simulink model "gm_Watermarker_vnl"  (R2022a)
settings: Solver=FixedStepDiscrete  StartTime=0.0  StopTime=256*256-1  RelTol=1e-3
undefined symbols (not defined in the file or in its folder): alpha, T0, T1
libraries: hdlsllib x20, simulink x2, dspsrcs4 x2
Description:
  | Performs watermarking.
  | In:
  | - One channel of 8-bit image 256x256
  | - Watermark (64 bits)
  | Out:
  | - Watermarked image channel
settings Model: SimulationMode=accelerator  Creator=The MathWorks, Inc.  LastModifiedBy=Администратор
settings SolverCC: AlgebraicLoopSolver=TrustRegion
settings DataIOCC: LimitDataPoints=on  SaveFormat=Structure  SaveTime=off  ReturnWorkspaceOutputs=off
settings OptimizationCC: BlockReduction=off  ConditionallyExecuteInputs=off  DefaultParameterBehavior=Inlined  InheritOutputTypeSmallerThanSingle=on  LifeSpan=inf
settings DebuggingCC: AlgebraicLoopMsg=error  UnderspecifiedInitializationDetection=Classic  MergeDetectMultiDrivingBlocksExec=none  SolverPrmCheckMsg=warning  InheritedTsInSrcMsg=none  SingleTaskRateTransMsg=error  ParameterPrecisionLossMsg=none  UnconnectedInputMsg=warning  UnconnectedOutputMsg=warning  UnconnectedLineMsg=warning  AllowSymbolicDim=off  SFUnexpectedBacktrackingDiag=warning  SFNoUnconditionalDefaultTransitionDiag=warning  SFExecutionAtInitializationDiag=none  SFMachineParentedDataDiag=warning  ArithmeticOperatorsInVariantConditions=warning
settings HardwareCC: ProdBitPerPointer=32  ProdBitPerSizeT=32  ProdBitPerPtrDiffT=32  ProdLargestAtomicFloat=None  ProdIntDivRoundTo=Undefined  ProdEndianess=Unspecified  ProdWordSize=32  ProdHWDeviceType=ASIC/FPGA->ASIC/FPGA  TargetBitPerPointer=64  TargetBitPerSizeT=64  TargetBitPerPtrDiffT=64  TargetLongLongMode=on  TargetIntDivRoundTo=Zero  TargetEndianess=LittleEndian  TargetWordSize=64  TargetHWDeviceType=Custom Processor->MATLAB Host Computer  ProdEqTarget=off
settings ModelReferenceCC: PropagateSignalLabelsOutOfModel=off
settings SFSimCC: SimUseLocalCustomCode=off  CustomCodeUndefinedFunction=UseInterfaceOnly
settings RTWCC: RTWUseLocalCustomCode=off  DLArmComputeVersion=19.05
settings CodeAppCC: StateflowObjectComments=on
settings GRTTargetCC: TargetLangStandard=C89/C90 (ANSI)
settings ConfigComp: CovMetricSettings=dw  CovSaveCumulativeToWorkspaceVar=on  CovSaveSingleToWorkspaceVar=on  CovExternalEMLEnable=off  CovSFcnEnable=off

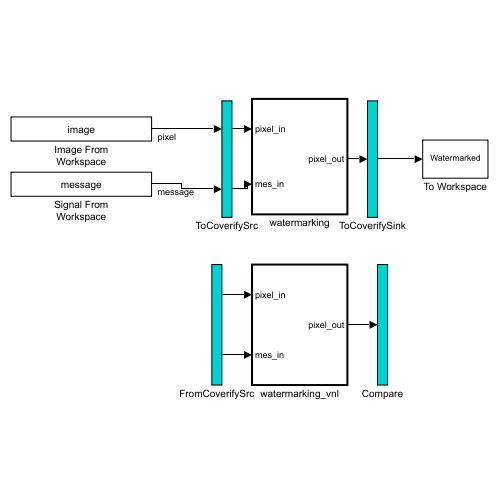
[thumbnail: Simulink's stored preview of the top-level diagram]
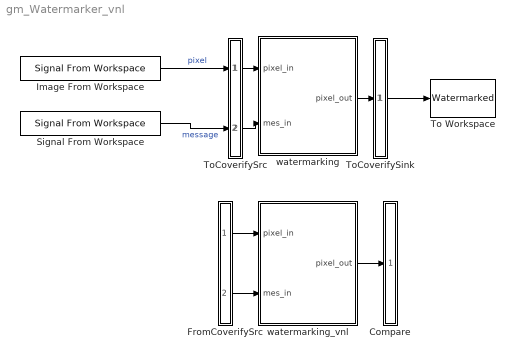
== system gm_Watermarker_vnl ==
  Compare : Subsystem
      mask Display: disp('')
  FromCoverifySrc : Subsystem
      mask Display: disp('')
  Image From Workspace : dspsrcs4/Signal From Workspace  X=image  Ts=1  nsamps=1  OutputAfterFinalValue=Cyclic repetition  ignoreOrWarnInputAndFrameLengths=off  OutputFrames=off
  Signal From Workspace : dspsrcs4/Signal From Workspace  X=message  Ts=1  nsamps=1  OutputAfterFinalValue=Cyclic repetition  ignoreOrWarnInputAndFrameLengths=off  OutputFrames=off
  To Workspace : ToWorkspace  VariableName=Watermarked  SampleTime=-1
      settings: Save2DSignal=2-D array (concatenate along first dimension)
  ToCoverifySink : Subsystem
      mask Display: disp('')
  ToCoverifySrc : Subsystem
      mask Display: disp('')
  watermarking : Subsystem  TreatAsAtomicUnit=on
  watermarking_vnl : Subsystem  TreatAsAtomicUnit=on
  wires:
  ToCoverifySrc/1(out1) -> watermarking/1(pixel_in)
  ToCoverifySrc/2(out2) -> watermarking/2(mes_in)
  watermarking/1(pixel_out) -> ToCoverifySink/1(in1)
  Image From Workspace/1 -> ToCoverifySrc/1(in1)  "pixel"
  Signal From Workspace/1 -> ToCoverifySrc/2(in2)  "message"
  ToCoverifySink/1(out1) -> To Workspace/1
  FromCoverifySrc/1(out1) -> watermarking_vnl/1(pixel_in)
  FromCoverifySrc/2(out2) -> watermarking_vnl/2(mes_in)
  watermarking_vnl/1(pixel_out) -> Compare/1(in1)

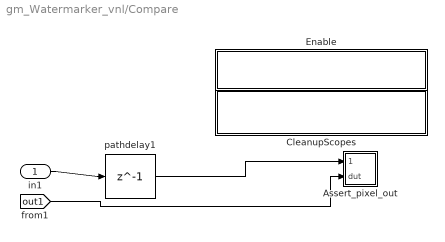
== system gm_Watermarker_vnl/Compare ==
  in1 : Inport
  Assert_pixel_out : Subsystem
  CleanupScopes : Subsystem
      settings: OpenFcn=|
      | blkName = gcb; %self block
      | idx = regexp(blkName, '/CleanupScopes$', 'once');
      | blkParent = blkName(1:idx-1);
      | blks=find_system(blkParent, 'LookUnderMasks', 'all','blocktype', 'Scope');
      | for itr = 1:length(blks)
      | 	 hScopeCfg = get_param(blks{itr},'ScopeConfiguration');
      | 	 hScopeCfg.Visible = ~ hScopeCfg.Visible;
      | end
      | drawnow;
      mask Display: fprintf(message('hdlcoder:cosim:vnl_dblclick').getString());
  Enable : Subsystem
      settings: OpenFcn=|
      | blkName = gcb;
      | idx = regexp(blkName, '/Enable$', 'once');
      | blkParent = blkName(1:idx-1);
      | blks=find_system(blkParent, 'LookUnderMasks', 'all','blocktype', 'Assertion');
      | e = get_param(blks{1}, 'Enabled');
      | if strcmp(e, 'on'), f= 'off';, else, f = 'on';, end
      | for ii=1:length(blks), set_param(blks{ii}, 'Enabled', f);, end
      | set_param(gcb, 'MaskDisplay',['fprintf(message(''hdlcoder:cosim:vnl_dblclick_assertions'',','''',upper(e),'''',').getString())']);
      mask Display: fprintf(message('hdlcoder:cosim:vnl_dblclick_assertions','OFF').getString());
  pathdelay1 : Delay  DelayLength=1
  wires:
  in1/1 -> pathdelay1/1
  pathdelay1/1 -> Assert_pixel_out/1(cosim)
  [out1] -> Assert_pixel_out/2(dut)

== system gm_Watermarker_vnl/FromCoverifySrc ==
  out1 : Outport
  out2 : Outport  Port=2
  wires:
  [in1] -> out1/1
  [in2] -> out2/1

== system gm_Watermarker_vnl/ToCoverifySink ==
  in1 : Inport
  out1 : Outport
  tag scope: out1=global
  wires:
  in1/1 -> out1/1, [out1]

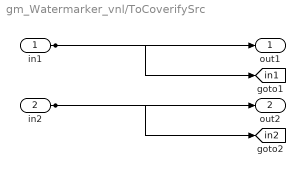
== system gm_Watermarker_vnl/ToCoverifySrc ==
  in1 : Inport
  in2 : Inport  Port=2
  out1 : Outport
  out2 : Outport  Port=2
  tag scope: in1=global, in2=global
  wires:
  in1/1 -> out1/1, [in1]
  in2/1 -> out2/1, [in2]

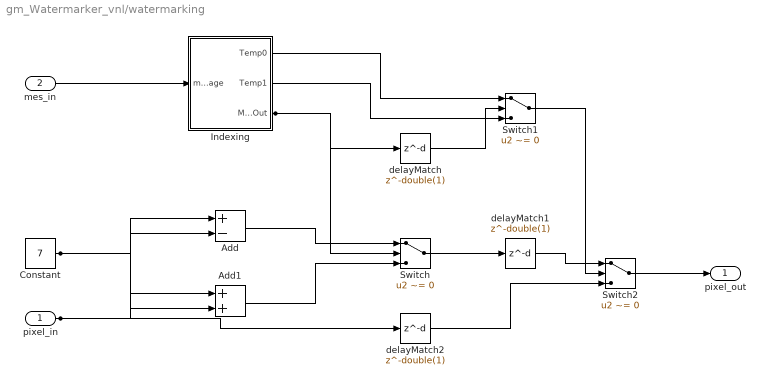
== system gm_Watermarker_vnl/watermarking ==
  pixel_in : Inport  OutDataTypeStr=uint8  PortDimensions=1  SampleTime=1
  mes_in : Inport  Port=2  OutDataTypeStr=boolean  PortDimensions=1  SampleTime=1
  Add : Sum  Inputs=+-  AccumDataTypeStr=uint8  OutDataTypeStr=uint8  SampleTime=1
  Add1 : Sum  AccumDataTypeStr=uint8  OutDataTypeStr=uint8  SampleTime=1
  Constant : Constant  Value=7  OutDataTypeStr=uint8  SampleTime=1
  Indexing : Subsystem
  Switch : Switch  Criteria=u2 ~= 0  Threshold=double(0)  OutDataTypeStr=uint8  SampleTime=1  SaturateOnIntegerOverflow=off  InputSameDT=off
  Switch1 : Switch  Criteria=u2 ~= 0  Threshold=double(0)  OutDataTypeStr=boolean  SampleTime=1  SaturateOnIntegerOverflow=off  InputSameDT=off
  Switch2 : Switch  Criteria=u2 ~= 0  Threshold=double(0)  OutDataTypeStr=uint8  SampleTime=1  SaturateOnIntegerOverflow=off  InputSameDT=off
  delayMatch : Delay  DelayLength=double(1)  InitialCondition=0  SampleTime=1
  delayMatch1 : Delay  DelayLength=double(1)  InitialCondition=0  SampleTime=1
  delayMatch2 : Delay  DelayLength=double(1)  InitialCondition=0  SampleTime=1
  pixel_out : Outport  SampleTime=1  VectorParamsAs1DForOutWhenUnconnected=off
  wires:
  pixel_in/1 -> Add/1, Add1/2, delayMatch2/1
  Switch/1 -> delayMatch1/1
  Indexing/3(MessageOut) -> Switch/2, delayMatch/1
  Switch2/1 -> pixel_out/1
  Switch1/1 -> Switch2/2
  delayMatch1/1 -> Switch2/1
  delayMatch/1 -> Switch1/2
  Indexing/2(Temp1) -> Switch1/3
  Indexing/1(Temp0) -> Switch1/1
  Constant/1 -> Add/2, Add1/1
  Add1/1 -> Switch/3
  Add/1 -> Switch/1
  mes_in/1 -> Indexing/1(message)
  delayMatch2/1 -> Switch2/3

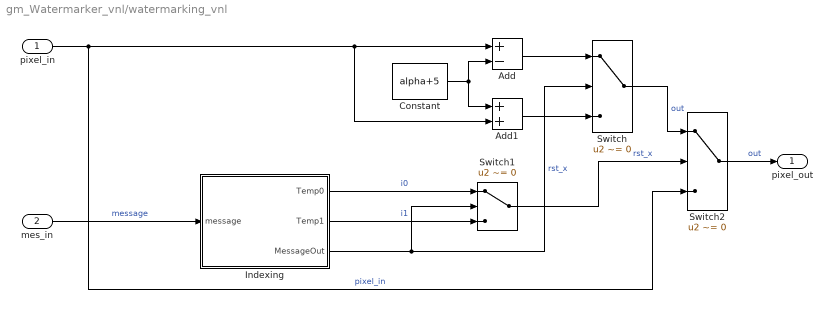
== system gm_Watermarker_vnl/watermarking_vnl ==
  pixel_in : Inport
  mes_in : Inport  Port=2
  Add : Sum  Inputs=+-  OutMin=[0]  OutMax=[255]  OutDataTypeStr=uint8
  Add1 : Sum  OutMin=[0]  OutMax=[255]  OutDataTypeStr=uint8
  Constant : Constant  Value=alpha+5  OutDataTypeStr=uint8  SampleTime=-1
  Indexing : Subsystem
  Switch : Switch  Criteria=u2 ~= 0  SaturateOnIntegerOverflow=off  InputSameDT=off
  Switch1 : Switch  Criteria=u2 ~= 0  SaturateOnIntegerOverflow=off  InputSameDT=off
  Switch2 : Switch  Criteria=u2 ~= 0  SaturateOnIntegerOverflow=off  InputSameDT=off
  pixel_out : Outport  VectorParamsAs1DForOutWhenUnconnected=off
  wires:
  Switch2/1 -> pixel_out/1  "out"
  Switch1/1 -> Switch2/2  "rst_x"
  Indexing/2(Temp1) -> Switch1/3  "i1"
  Indexing/1(Temp0) -> Switch1/1  "i0"
  Switch/1 -> Switch2/1  "out"
  Add1/1 -> Switch/3
  Add/1 -> Switch/1
  Constant/1 -> Add/2, Add1/1
  pixel_in/1 -> Switch2/3, Add/1, Add1/2  "pixel_in"
  Indexing/3(MessageOut) -> Switch/2, Switch1/2  "rst_x"
  mes_in/1 -> Indexing/1(message)  "message"

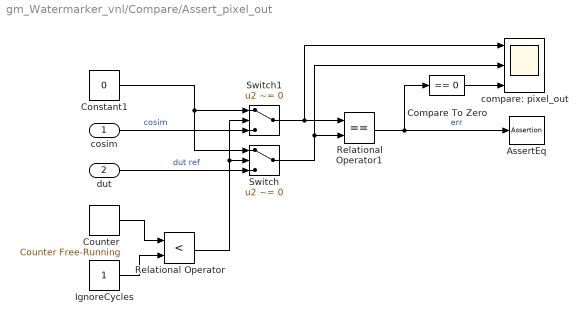
== system gm_Watermarker_vnl/Compare/Assert_pixel_out ==
  cosim : Inport
  dut : Inport  Port=2
  AssertEq : Assertion  StopWhenAssertionFail=off
  Compare To Zero : simulink/Logic and Bit Operations/Compare To Zero  relop===  OutDataTypeStr=boolean
  Constant1 : Constant  Value=0  OutDataTypeStr=Inherit: Inherit via back propagation  SampleTime=-1
  Counter : simulink/Sources/Counter Free-Running  NumBits=32  tsamp=-1
  IgnoreCycles : Constant  OutDataTypeStr=Inherit: Inherit via back propagation  SampleTime=-1
  Relational Operator : RelationalOperator  Operator=<  OutDataTypeStr=boolean  InputSameDT=off
  Relational Operator1 : RelationalOperator  Operator===  OutDataTypeStr=boolean  InputSameDT=off
  Switch : Switch  Criteria=u2 ~= 0  SaturateOnIntegerOverflow=off  InputSameDT=off
  Switch1 : Switch  Criteria=u2 ~= 0  SaturateOnIntegerOverflow=off  InputSameDT=off
  compare: pixel_out : Scope  NumInputPorts=3
  wires:
  Compare To Zero/1 -> compare: pixel_out/3
  Relational Operator1/1 -> Compare To Zero/1, AssertEq/1  "err"
  Switch1/1 -> compare: pixel_out/1, Relational Operator1/1
  Switch/1 -> compare: pixel_out/2, Relational Operator1/2
  Constant1/1 -> Switch/1, Switch1/1
  Relational Operator/1 -> Switch/2, Switch1/2
  cosim/1 -> Switch1/3  "cosim"
  dut/1 -> Switch/3  "dut ref"
  Counter/1 -> Relational Operator/1
  IgnoreCycles/1 -> Relational Operator/2

== system gm_Watermarker_vnl/Compare/CleanupScopes ==

== system gm_Watermarker_vnl/Compare/Enable ==

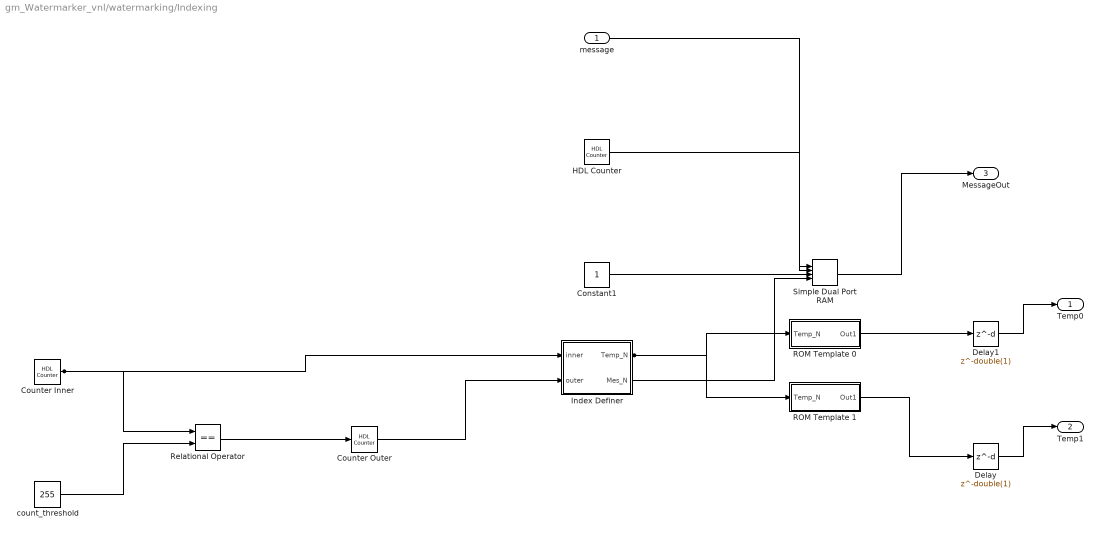
== system gm_Watermarker_vnl/watermarking/Indexing ==
  message : Inport  OutDataTypeStr=boolean  PortDimensions=1  SampleTime=1
  Constant1 : Constant  OutDataTypeStr=boolean  SampleTime=1
  Counter Inner : hdlsllib/Sources/HDL Counter  CountType=Count limited  CountInit=0  CountStep=1  CountMax=255  CountFromType=Initial value  CountFrom=0  CountResetPort=off  CountLoadPort=off  CountEnbPort=off  CountDirPort=off  CountHitOutputPort=off  CountDataType=Unsigned  CountWordLen=8  CountFracLen=0  CountSampTime=1
  Counter Outer : hdlsllib/Sources/HDL Counter  CountType=Count limited  CountInit=0  CountStep=1  CountMax=255  CountFromType=Initial value  CountFrom=0  CountResetPort=off  CountLoadPort=off  CountEnbPort=on  CountDirPort=off  CountHitOutputPort=off  CountDataType=Unsigned  CountWordLen=8  CountFracLen=0  CountSampTime=1
  Delay : Delay  DelayLength=double(1)  InitialCondition=0  SampleTime=1
  Delay1 : Delay  DelayLength=double(1)  InitialCondition=0  SampleTime=1
  HDL Counter : hdlsllib/Sources/HDL Counter  CountType=Count limited  CountInit=0  CountStep=1  CountMax=63  CountFromType=Initial value  CountFrom=0  CountResetPort=off  CountLoadPort=off  CountEnbPort=off  CountDirPort=off  CountHitOutputPort=off  CountDataType=Unsigned  CountWordLen=6  CountFracLen=0  CountSampTime=1
  Index Definer : Subsystem
  ROM Template 0 : Subsystem
  ROM Template 1 : Subsystem
  Relational Operator : RelationalOperator  Operator===  OutDataTypeStr=boolean  SampleTime=1  InputSameDT=off
  Simple Dual Port RAM : hdlsllib/HDL RAMs/Simple Dual Port RAM  ram_size=6
      settings: SourceProductBaseCode=SL
  count_threshold : Constant  Value=255  OutDataTypeStr=uint8  SampleTime=1
  Temp0 : Outport  SampleTime=1
  Temp1 : Outport  Port=2  SampleTime=1
  MessageOut : Outport  Port=3  SampleTime=1
  wires:
  message/1 -> Simple Dual Port RAM/1
  count_threshold/1 -> Relational Operator/2
  Simple Dual Port RAM/1 -> MessageOut/1
  Relational Operator/1 -> Counter Outer/1
  ROM Template 1/1(Out1) -> Delay/1
  ROM Template 0/1(Out1) -> Delay1/1
  Index Definer/2(Mes_N) -> Simple Dual Port RAM/4
  Index Definer/1(Temp_N) -> ROM Template 1/1(Temp_N), ROM Template 0/1(Temp_N)
  HDL Counter/1 -> Simple Dual Port RAM/2
  Delay1/1 -> Temp0/1
  Delay/1 -> Temp1/1
  Counter Outer/1 -> Index Definer/2(outer)
  Counter Inner/1 -> Index Definer/1(inner), Relational Operator/1
  Constant1/1 -> Simple Dual Port RAM/3

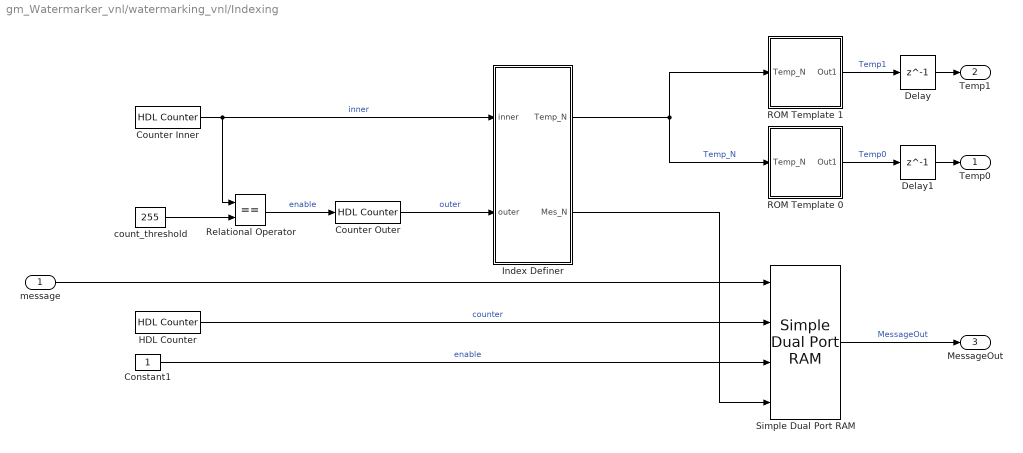
== system gm_Watermarker_vnl/watermarking_vnl/Indexing ==
  message : Inport
  Constant1 : Constant  OutMin=[1]  OutMax=[1]  OutDataTypeStr=boolean  SampleTime=-1
  Counter Inner : hdlsllib/Sources/HDL Counter  CountType=Count limited  CountInit=0  CountStep=1  CountMax=255  CountFromType=Initial value  CountFrom=0  CountResetPort=off  CountLoadPort=off  CountEnbPort=off  CountDirPort=off  CountHitOutputPort=off  CountDataType=Unsigned  CountWordLen=8  CountFracLen=0  CountSampTime=1
  Counter Outer : hdlsllib/Sources/HDL Counter  CountType=Count limited  CountInit=0  CountStep=1  CountMax=255  CountFromType=Initial value  CountFrom=0  CountResetPort=off  CountLoadPort=off  CountEnbPort=on  CountDirPort=off  CountHitOutputPort=off  CountDataType=Unsigned  CountWordLen=8  CountFracLen=0  CountSampTime=1
  Delay : Delay  DelayLength=1  InitialCondition=0
  Delay1 : Delay  DelayLength=1  InitialCondition=0
  HDL Counter : hdlsllib/Sources/HDL Counter  CountType=Count limited  CountInit=0  CountStep=1  CountMax=63  CountFromType=Initial value  CountFrom=0  CountResetPort=off  CountLoadPort=off  CountEnbPort=off  CountDirPort=off  CountHitOutputPort=off  CountDataType=Unsigned  CountWordLen=6  CountFracLen=0  CountSampTime=1
  Index Definer : Subsystem
  ROM Template 0 : Subsystem
  ROM Template 1 : Subsystem
  Relational Operator : RelationalOperator  Operator===  OutDataTypeStr=boolean  InputSameDT=off
  Simple Dual Port RAM : hdlsllib/HDL RAMs/Simple Dual Port RAM  ram_size=6
      settings: SourceProductBaseCode=SL
  count_threshold : Constant  Value=255  OutMin=[255]  OutMax=[255]  OutDataTypeStr=uint8  SampleTime=-1
  Temp0 : Outport
  Temp1 : Outport  Port=2
  MessageOut : Outport  Port=3
  wires:
  Delay1/1 -> Temp0/1
  Delay/1 -> Temp1/1
  message/1 -> Simple Dual Port RAM/1
  ROM Template 1/1(Out1) -> Delay/1  "Temp1"
  ROM Template 0/1(Out1) -> Delay1/1  "Temp0"
  Index Definer/1(Temp_N) -> ROM Template 1/1(Temp_N), ROM Template 0/1(Temp_N)  "Temp_N"
  Index Definer/2(Mes_N) -> Simple Dual Port RAM/4
  Counter Outer/1 -> Index Definer/2(outer)  "outer"
  Constant1/1 -> Simple Dual Port RAM/3  "enable"
  Relational Operator/1 -> Counter Outer/1  "enable"
  Simple Dual Port RAM/1 -> MessageOut/1  "MessageOut"
  count_threshold/1 -> Relational Operator/2
  Counter Inner/1 -> Relational Operator/1, Index Definer/1(inner)  "inner"
  HDL Counter/1 -> Simple Dual Port RAM/2  "counter"

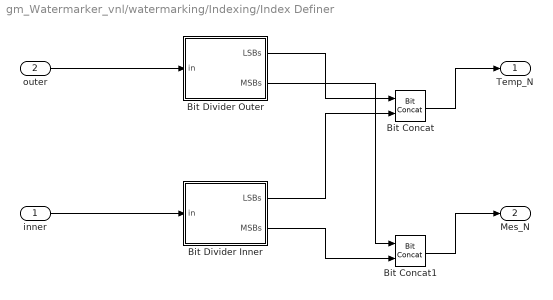
== system gm_Watermarker_vnl/watermarking/Indexing/Index Definer ==
  inner : Inport  OutDataTypeStr=uint8  PortDimensions=1  SampleTime=1
  outer : Inport  Port=2  OutDataTypeStr=uint8  PortDimensions=1  SampleTime=1
  Bit Concat : hdlsllib/Logic and Bit Operations/Bit Concat  numInputs=2
  Bit Concat1 : hdlsllib/Logic and Bit Operations/Bit Concat  numInputs=2
  Bit Divider Inner : Subsystem
  Bit Divider Outer : Subsystem
  Temp_N : Outport  SampleTime=1
  Mes_N : Outport  Port=2  SampleTime=1
  wires:
  outer/1 -> Bit Divider Outer/1(in)
  inner/1 -> Bit Divider Inner/1(in)
  Bit Divider Outer/2(MSBs) -> Bit Concat1/1
  Bit Divider Outer/1(LSBs) -> Bit Concat/1
  Bit Divider Inner/2(MSBs) -> Bit Concat1/2
  Bit Divider Inner/1(LSBs) -> Bit Concat/2
  Bit Concat1/1 -> Mes_N/1
  Bit Concat/1 -> Temp_N/1

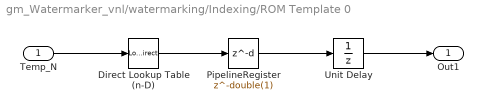
== system gm_Watermarker_vnl/watermarking/Indexing/ROM Template 0 ==
  Temp_N : Inport  OutDataTypeStr=fixdt(0, 10, 0)  PortDimensions=1  SampleTime=1
  Direct Lookup Table (n-D) : LookupNDDirect  NumberOfTableDimensions=1  Table="reshape(logical([1 1 1 0 0 0 0 0 1 1 1 0 0 0 0 0 0 0 0 0 0 1 1 1 0 0 0 0 0 1 1 1 1 1 0 0 0 0 0 0 0 0 1 1 1 0 0 0 0 0 0 0 1 1 0 0 0 0 0 0 0 0 0 1 0 0 0 0 0 0 0 0 0 0 0 1 1 1 0 0 0 0 1 1 1 0 0 0 0 0 0 0 0 0 0 0 0 0 0 0 0 0 0 0 0 0 0 0 0 1 1 1 1 1 1 1 0 0 0 0 0 0 0 0 0 0 0 0 0 0 0 0 0 0 0 0 0 0 0 0 0 0 1 1 1 1 0 0 0 0 0 0 0 0 0 0 0 0 0 0 0 0 0 0 0 0 0 0 0 0 0 0 0 0 0 0 0 0 0 0 0 0 0 0 0 0 0 0 0 0 0 0 0 0 0 1 1 1 1 1 1 0 0 0 0 0 0 0 0 0 0 0 0 0 0 0 1 1 1 1 1 0 0 0 0 1 1 1 1 1 1 1 1 1 0 0 0 0 0 0 0 0 0 0 0 0 1 1 1 1 1 1 1 1 1 0 1 1 1 0 0 0 0 0 0 1 1 0 0 0 0 0 0 0 0 0 0 1 1 1 0 0 0 0 0 1 1 1 1 0 0 0 0 0 0 0 0 0 1 1 1 0 0 0 0 0 0 0 1 1 0 0 0 0 0 0 0 0 0 1 0 0 0 0 0 0 0 0 0 0 0 1 1 1 0 0 0 0 1 1 1 0 0 0 0 0 0 0 0 0 0 0 0 0 0 0 0 0 0 0 0 0 0 0 0 1 1 1 1 1 1 1 0 0 0 0 0 0 0 0 0 0 0 0 0 0 0 0 0 0 0 0 0 0 0 0 0 0 1 1 1 1 0 0 0 0 0 0 0 0 0 0 0 0 0 0 0 0 0 0 0 1 1 1 0 0 0 0 0 0 0 0 0 0 0 0 0 0 0 0 0 0 1 1 1 0 0 0 0 0 0 1 1 1 1 1 1 0 0 0 0 0 0 0 0 0 0 0 0 0 0 0 1 1 1 1 1 1 0 0 0 1 1 1 1 0 1 1 1 1 0 0 0 0 0 0 0 0 0 0 0 0 1 1 1 1 0 1 1 1 1 0 1 1 1 0 0 0 0 0 0 1 1 0 0 0 0 0 0 0 0 0 0 1 1 1 0 0 0 0 0 1 1 1 1 0 0 0 0 0 0 0 0 0 1 1 1 0 0 0 0 0 0 1 1 1 0 0 0 0 0 0 0 0 0 1 0 0 0 0 0 0 0 0 0 0 0 1 1 1 0 0 0 0 1 1 1 0 0 0 0 0 0 0 0 0 0 0 0 0 0 0 0 0 0 0 0 0 0 0 0 1 1 1 1 1 1 0 0 0 0 0 0 0 0 0 0 0 0 0 0 0 0 0 0 0 0 0 0 0 0 0 0 0 1 1 1 1 0 0 0 0 0 0 0 0 0 0 0 0 0 0 0 0 0 0 0 1 1 1 0 0 0 0 0 0 0 0 0 0 0 0 0 0 0 0 0 1 1 1 0 0 0 0 0 0 0 1 1 1 1 1 1 0 0 0 0 0 0 0 0 0 0 0 0 0 0 0 1 1 1 1 1 1 0 0 0 1 1 1 1 0 1 1 1 1 0 0 0 0 0 0 0 0 0 0 0 0 1 1 1 1 0 1 1 1 1 0 1 1 1 0 0 0 0 0 0 1 1 0 0 0 0 0 0 0 0 0 0 1 1 1 0 0 0 0 0 0 1 1 1 0 0 0 0 0 0 0 0 0 1 1 1 0 0 0 0 0 0 1 1 1 0 0 0 0 0 0 0 0 0 1 0 0 0 0 0 0 0 0 0 0 0 1 1 1 1 0 0 0 1 1 1 0 0 0 0 0 0 0 0 0 0 0 0 0 0 0 0 0 0 0 0 0 0 0 0 1 1 1 1 1 1 1 0 0 0 0 0 0 0 0 0 0 0 0 0 0 0 0 0 0 0 0 0 0 0 0 0 0 1 1 1 1 0 0 0 0 0 0 0 0 0 0 0 0 0 0 0 0 0 0 0 1 1 0 0 0 0 0 0 0 0 0 0 0 0 0 0 0 0 0 0 0 1 1 0 0 0 0 0 0 0 1 1 1 1 1 1 0 0 0 0 0 0 0 0 0 0 0 0 0 0 1 1 1 1 1 1 1 0 0 0 1 1 1 1 0 1 1 1 1 0 0 0 0 0 0 0 0 0 0 0 0 1 1 1 1 0 0 1 1 1 0]).', [1024     1])"  DiagnosticForOutOfRangeInput=Error  SampleTime=1  TableDataTypeStr=boolean
  PipelineRegister : Delay  DelayLength=double(1)  InitialCondition=0  SampleTime=1
  Unit Delay : UnitDelay  SampleTime=1
  Out1 : Outport  SampleTime=1
  wires:
  Direct Lookup Table (n-D)/1 -> PipelineRegister/1
  Temp_N/1 -> Direct Lookup Table (n-D)/1
  Unit Delay/1 -> Out1/1
  PipelineRegister/1 -> Unit Delay/1

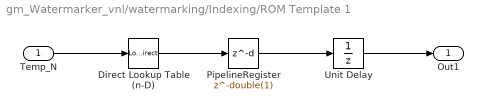
== system gm_Watermarker_vnl/watermarking/Indexing/ROM Template 1 ==
  Temp_N : Inport  OutDataTypeStr=fixdt(0, 10, 0)  PortDimensions=1  SampleTime=1
  Direct Lookup Table (n-D) : LookupNDDirect  NumberOfTableDimensions=1  Table="reshape(logical([1 1 0 0 0 0 0 0 0 0 0 1 1 1 0 0 0 0 0 0 1 1 0 0 0 0 0 0 0 0 0 0 1 1 1 0 0 0 0 0 0 0 1 1 1 0 0 0 0 0 0 0 0 1 1 1 0 0 0 0 0 0 0 1 0 1 1 1 1 0 0 0 1 1 1 0 0 0 0 0 0 0 0 0 0 0 1 1 1 1 0 0 0 1 1 1 0 0 0 1 1 1 1 1 1 1 0 0 0 0 0 0 0 0 0 0 0 0 0 0 1 1 1 1 1 1 1 0 0 0 0 0 0 1 1 1 0 0 0 0 0 0 0 0 0 0 0 0 0 0 0 0 0 0 1 1 1 0 0 0 0 0 0 0 0 0 0 0 0 0 0 0 0 0 0 0 1 1 0 0 0 0 0 0 0 0 0 0 0 0 0 0 0 0 0 0 0 0 0 0 0 0 0 0 0 0 1 1 1 1 1 1 0 0 0 0 0 0 0 0 0 0 0 0 0 0 0 0 0 0 0 0 0 0 0 0 1 1 1 1 1 1 1 1 1 0 0 0 0 0 0 0 0 0 0 0 1 1 0 0 0 0 0 0 0 0 0 1 1 1 1 0 0 0 0 1 1 1 0 0 0 0 0 0 0 0 0 0 1 1 1 0 0 0 0 0 0 0 1 1 1 0 0 0 0 0 0 0 0 1 1 1 0 0 0 0 0 0 0 1 0 1 1 1 1 0 0 0 1 1 1 0 0 0 0 0 0 0 0 0 0 0 1 1 1 1 0 0 0 1 1 1 0 0 0 1 1 1 1 1 1 1 0 0 0 0 0 0 0 0 0 0 0 0 0 0 1 1 1 1 1 1 1 0 0 0 0 0 0 1 1 1 0 0 0 0 0 0 0 0 0 0 0 0 0 0 0 0 0 1 1 1 1 0 0 0 0 0 0 0 0 0 0 0 0 0 0 0 0 0 0 0 1 1 0 0 0 0 0 0 0 0 0 0 0 0 0 0 0 0 0 0 0 0 0 0 0 0 0 0 0 0 1 1 1 1 1 1 0 0 0 0 0 0 0 0 0 0 0 0 0 0 0 0 0 0 0 0 0 0 0 0 1 1 1 1 1 1 1 1 1 0 0 0 0 0 0 0 0 0 0 0 1 1 0 0 0 0 0 0 0 0 0 1 1 1 1 0 0 0 0 1 1 1 0 0 0 0 0 0 0 0 0 0 1 1 1 0 0 0 0 0 0 0 1 1 0 0 0 0 0 0 0 0 0 1 1 1 0 0 0 0 0 0 0 1 0 0 1 1 1 0 0 0 1 1 1 0 0 0 0 0 0 0 0 0 0 0 1 1 1 1 0 0 0 1 1 1 0 0 0 1 1 1 1 1 1 1 0 0 0 0 0 0 0 0 0 0 0 0 0 0 1 1 1 1 1 1 1 0 0 0 0 0 0 1 1 1 0 0 0 0 0 0 0 0 0 0 0 0 0 0 0 0 0 0 1 1 1 0 0 0 0 0 0 0 0 0 0 0 0 0 0 0 0 0 0 0 1 1 0 0 0 0 0 0 0 0 0 0 0 0 0 0 0 0 0 0 0 0 0 0 0 0 0 0 0 0 1 1 1 1 1 1 0 0 0 0 0 0 0 0 0 0 0 0 0 0 0 0 0 0 0 0 0 0 0 0 1 1 1 1 1 1 1 1 1 0 0 0 0 0 0 0 0 0 0 0 1 1 0 0 0 0 0 0 0 0 0 1 1 1 1 0 0 0 0 1 1 1 1 0 0 0 0 0 0 0 0 0 1 1 1 0 0 0 0 0 0 0 1 1 0 0 0 0 0 0 0 0 0 1 1 1 0 0 0 0 0 0 0 1 0 0 1 1 1 0 0 0 1 1 1 0 0 0 0 0 0 0 0 0 0 0 0 1 1 1 0 0 0 1 1 1 0 0 0 1 1 1 1 1 1 1 0 0 0 0 0 0 0 0 0 0 0 0 0 0 1 1 1 1 1 1 1 0 0 0 0 0 0 1 1 1 0 0 0 0 0 0 0 0 0 0 0 0 0 0 0 0 0 0 1 1 1 0 0 0 0 0 0 0 0 0 0 0 0 0 0 0 0 0 0 0 0 0 0 0 0 0 0 0 0 0 0 0 0 0 0 0 0 0 0 0 0 0 0 0 0 0 0 0 0 0 1 1 1 1 1 1 0 0 0 0 0 0 0 0 0 0 0 0 0 0 0 0 0 0 0 0 0 0 0 0 1 1 1 1 0 1 1 1 1 0 0 0 0 0 0 0 0 0 0 0]).', [1024     1])"  DiagnosticForOutOfRangeInput=Error  SampleTime=1  TableDataTypeStr=boolean
  PipelineRegister : Delay  DelayLength=double(1)  InitialCondition=0  SampleTime=1
  Unit Delay : UnitDelay  SampleTime=1
  Out1 : Outport  SampleTime=1
  wires:
  Direct Lookup Table (n-D)/1 -> PipelineRegister/1
  Temp_N/1 -> Direct Lookup Table (n-D)/1
  Unit Delay/1 -> Out1/1
  PipelineRegister/1 -> Unit Delay/1

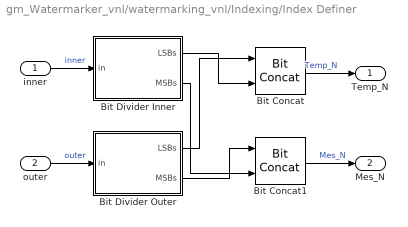
== system gm_Watermarker_vnl/watermarking_vnl/Indexing/Index Definer ==
  inner : Inport
  outer : Inport  Port=2
  Bit Concat : hdlsllib/Logic and Bit Operations/Bit Concat  numInputs=2
  Bit Concat1 : hdlsllib/Logic and Bit Operations/Bit Concat  numInputs=2
  Bit Divider Inner : Subsystem
  Bit Divider Outer : Subsystem
  Temp_N : Outport
  Mes_N : Outport  Port=2
  wires:
  Bit Divider Outer/1(LSBs) -> Bit Concat/1
  Bit Divider Inner/2(MSBs) -> Bit Concat1/2
  Bit Divider Outer/2(MSBs) -> Bit Concat1/1
  inner/1 -> Bit Divider Inner/1(in)  "inner"
  Bit Concat1/1 -> Mes_N/1  "Mes_N"
  Bit Concat/1 -> Temp_N/1  "Temp_N"
  Bit Divider Inner/1(LSBs) -> Bit Concat/2
  outer/1 -> Bit Divider Outer/1(in)  "outer"

== system gm_Watermarker_vnl/watermarking_vnl/Indexing/ROM Template 0 ==
  Temp_N : Inport
  Direct Lookup Table (n-D) : LookupNDDirect  NumberOfTableDimensions=1  Table=T0  DiagnosticForOutOfRangeInput=Error  TableMin=[0]  TableMax=[1]
  Unit Delay : UnitDelay  SampleTime=-1  HasFrameUpgradeWarning=on
  Out1 : Outport
  wires:
  Direct Lookup Table (n-D)/1 -> Unit Delay/1
  Temp_N/1 -> Direct Lookup Table (n-D)/1
  Unit Delay/1 -> Out1/1

== system gm_Watermarker_vnl/watermarking_vnl/Indexing/ROM Template 1 ==
  Temp_N : Inport
  Direct Lookup Table (n-D) : LookupNDDirect  NumberOfTableDimensions=1  Table=T1  DiagnosticForOutOfRangeInput=Error  TableMin=[0]  TableMax=[1]
  Unit Delay : UnitDelay  SampleTime=-1  HasFrameUpgradeWarning=on
  Out1 : Outport
  wires:
  Direct Lookup Table (n-D)/1 -> Unit Delay/1
  Temp_N/1 -> Direct Lookup Table (n-D)/1
  Unit Delay/1 -> Out1/1

== system gm_Watermarker_vnl/watermarking/Indexing/Index Definer/Bit Divider Inner ==
  in : Inport  OutDataTypeStr=uint8  PortDimensions=1  SampleTime=1
  Bit Slice : hdlsllib/Logic and Bit Operations/Bit Slice  lidx=double(4)  ridx=double(0)
      settings: SourceProductBaseCode=SL
  Bit Slice1 : hdlsllib/Logic and Bit Operations/Bit Slice  lidx=double(7)  ridx=double(5)
      settings: SourceProductBaseCode=SL
  LSBs : Outport  SampleTime=1
  MSBs : Outport  Port=2  SampleTime=1
  wires:
  in/1 -> Bit Slice/1, Bit Slice1/1
  Bit Slice1/1 -> MSBs/1
  Bit Slice/1 -> LSBs/1

== system gm_Watermarker_vnl/watermarking/Indexing/Index Definer/Bit Divider Outer ==
  in : Inport  OutDataTypeStr=uint8  PortDimensions=1  SampleTime=1
  Bit Slice : hdlsllib/Logic and Bit Operations/Bit Slice  lidx=double(4)  ridx=double(0)
      settings: SourceProductBaseCode=SL
  Bit Slice1 : hdlsllib/Logic and Bit Operations/Bit Slice  lidx=double(7)  ridx=double(5)
      settings: SourceProductBaseCode=SL
  LSBs : Outport  SampleTime=1
  MSBs : Outport  Port=2  SampleTime=1
  wires:
  in/1 -> Bit Slice/1, Bit Slice1/1
  Bit Slice1/1 -> MSBs/1
  Bit Slice/1 -> LSBs/1

== system gm_Watermarker_vnl/watermarking_vnl/Indexing/Index Definer/Bit Divider Inner ==
  in : Inport
  Bit Slice : hdlsllib/Logic and Bit Operations/Bit Slice  lidx=4  ridx=0
      settings: SourceProductBaseCode=SL
  Bit Slice1 : hdlsllib/Logic and Bit Operations/Bit Slice  lidx=7  ridx=5
      settings: SourceProductBaseCode=SL
  LSBs : Outport
  MSBs : Outport  Port=2
  wires:
  Bit Slice1/1 -> MSBs/1  "MSBs"
  Bit Slice/1 -> LSBs/1  "LSBs"
  in/1 -> Bit Slice1/1, Bit Slice/1  "inner"

== system gm_Watermarker_vnl/watermarking_vnl/Indexing/Index Definer/Bit Divider Outer ==
  in : Inport
  Bit Slice : hdlsllib/Logic and Bit Operations/Bit Slice  lidx=4  ridx=0
      settings: SourceProductBaseCode=SL
  Bit Slice1 : hdlsllib/Logic and Bit Operations/Bit Slice  lidx=7  ridx=5
      settings: SourceProductBaseCode=SL
  LSBs : Outport
  MSBs : Outport  Port=2
  wires:
  Bit Slice1/1 -> MSBs/1  "MSBs"
  Bit Slice/1 -> LSBs/1  "LSBs"
  in/1 -> Bit Slice1/1, Bit Slice/1  "outer"
